simulink model "HIL"  (R2022b)
settings: Solver=VariableStepAuto  StartTime=0.0  StopTime=60  RelTol=1e-3
undefined symbols (not defined in the file): LF
libraries: instrumentseriallib x3, etargetslib x1, dspfdesign x1
settings Model: Creator=eic20nr  LastModifiedBy=nikilesh
settings ModelReferenceCC: EnableRefExpFcnMdlSchedulingChecks=on

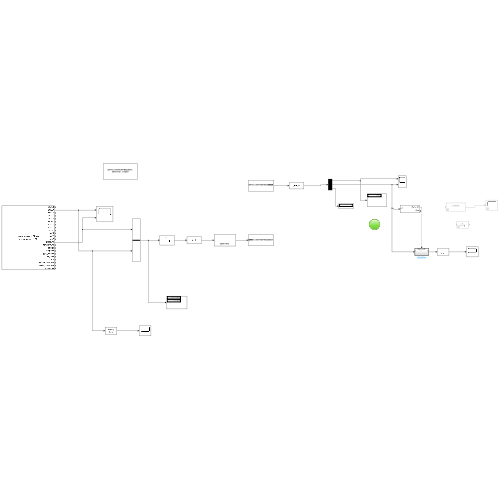
[thumbnail: Simulink's stored preview of the top-level diagram]
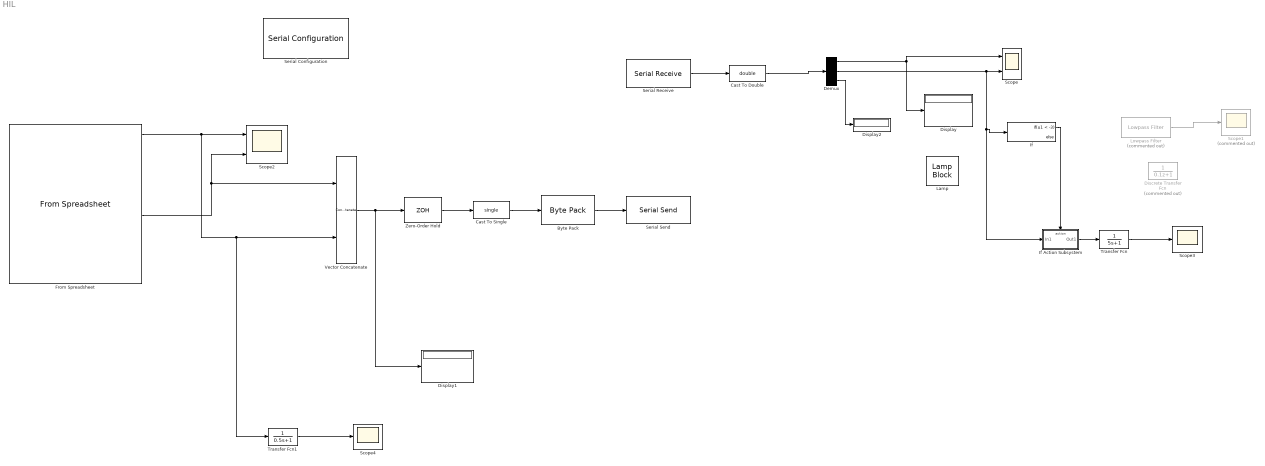
== system HIL ==
  Byte Pack : etargetslib/Byte Pack  datatypes={'single'}  byteAlign=4
  Cast To Double : DataTypeConversion  OutDataTypeStr=double  SaturateOnIntegerOverflow=off  RndMeth=Floor
  Cast To Single : DataTypeConversion  OutDataTypeStr=single  SaturateOnIntegerOverflow=off  RndMeth=Floor
  Demux : Demux  Outputs=3
  Discrete Transfer Fcn : DiscreteTransferFcn  Commented=on  Denominator=[0.1 1]
  Display : Display
  Display1 : Display
  Display2 : Display
  From Spreadsheet : FromSpreadsheet  FileName=march_launch_1_SF.xlsx  SheetName=march_launch_1_SF  SampleTime=0.05
  If : If  IfExpression=u1 < -3
  If Action Subsystem : Subsystem  TreatAsAtomicUnit=on
  Lamp : LampBlock  LabelPosition=Hide
  Lowpass Filter : dspfdesign/Lowpass Filter  Commented=on  FilterType=FIR  DesignForMinimumOrder=on  FilterOrder=50  PassbandFrequency=8e3  StopbandFrequency=12e3  PassbandRipple=0.1  StopbandAttenuation=80  InheritSampleRate=off  SampleRate=44100  SimulateUsing=Interpreted execution  roundingMode=Floor  coeffsDataTypeStr=fixdt(1,16)
  Scope : Scope  NumInputPorts=2
  Scope1 : Scope  Commented=on
  Scope2 : Scope  NumInputPorts=2
  Scope3 : Scope
  Scope4 : Scope
  Serial Configuration : instrumentseriallib/Serial Configuration  Priority=-200000  PortSel=/dev/cu.usbmodem83209501  Port=/dev/cu.usbmodem83209501  ComPort=/dev/cu.usbmodem83209501  BaudRate=115200  DataBits=8  Parity=none  StopBits=1  ByteOrder=little-endian  FlowControl=none  Timeout=10  SimulateUsing=Interpreted execution  BlockInModel=on  aMode=1
  Serial Receive : instrumentseriallib/Serial Receive  Priority=1  PortSel=/dev/cu.usbmodem83209501  Port=/dev/cu.usbmodem83209501  ComPort=/dev/cu.usbmodem83209501  DataType=single  SaveDataType=uint8  ToggleHeader=on  Header='A'  ToggleTerminator=on  Terminator=LF ('\n')  CustomTerminator=[]  InputFormat=Column major  ToggleDataSize=on  DataSize=[1 3]  EnableBlockingMode=on  ActionDataUnavailable=Output last received value  ActionWhenDataUnavailable=Output last received value  CustomValue=0  SampleTime=0.05  SimulateUsing=Interpreted execution  BlockInModel=on  aMode=1
  Serial Send : instrumentseriallib/Serial Send  Priority=1  PortSel=/dev/cu.usbmodem83209501  Port=/dev/cu.usbmodem83209501  ComPort=/dev/cu.usbmodem83209501  Header=[]  Terminator=<none>  CustomTerminator=[]  EnableBlockingMode=on  SimulateUsing=Interpreted execution  BlockInModel=on  aMode=1
  Transfer Fcn : TransferFcn  Denominator=[5 1]
  Transfer Fcn1 : TransferFcn  Denominator=[0.5 1]
  Vector Concatenate : Concatenate
  Zero-Order Hold : ZeroOrderHold  SampleTime=0.05
  wires:
  Serial Receive/1 -> Cast To Double/1
  Cast To Double/1 -> Demux/1
  Zero-Order Hold/1 -> Cast To Single/1
  Cast To Single/1 -> Byte Pack/1
  Byte Pack/1 -> Serial Send/1
  Vector Concatenate/1 -> Zero-Order Hold/1, Display1/1
  Demux/1 -> Scope/1, Display/1
  Demux/2 -> If/1, If Action Subsystem/1(In1), Scope/2
  From Spreadsheet/2 -> Transfer Fcn1/1, Vector Concatenate/2, Scope2/1
  Demux/3 -> Display2/1
  Lowpass Filter/1 -> Scope1/1
  Transfer Fcn/1 -> Scope3/1
  Transfer Fcn1/1 -> Scope4/1
  From Spreadsheet/13 -> Vector Concatenate/1, Scope2/2
  If Action Subsystem/1(Out1) -> Transfer Fcn/1
  If/1 -> If Action Subsystem/Action

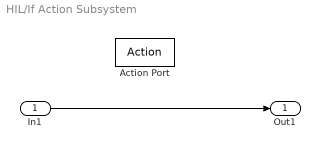
== system HIL/If Action Subsystem ==
  In1 : Inport
  Action Port : ActionPort  ActionPortLabel=if(u1 < -3)
  Out1 : Outport
  wires:
  In1/1 -> Out1/1
